simulink model "DANIEL_OLSSON_LAB10_stepX"  (R2021a)
settings: Solver=VariableStepAuto  StartTime=0.0  StopTime=10.0  RelTol=1e-3
settings Model: Creator=dmols  LastModifiedBy=dmols

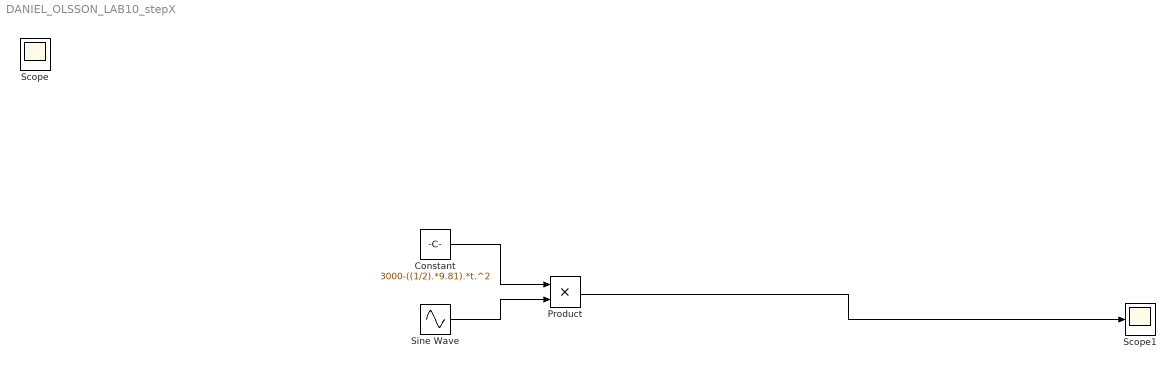
== system DANIEL_OLSSON_LAB10_stepX ==
  Constant : Constant  Value=3000-((1/2).*9.81).*t.^2  VectorParams1D=off
  Product : Product
  Scope1 : Scope
  Sine Wave : Sin  SampleTime=0
  Scope : Scope
  wires:
  Constant/1 -> Product/1
  Sine Wave/1 -> Product/2
  Product/1 -> Scope1/1
